simulink model "Wind_Turbine_MPPT_Simulation"  (R2023a)
settings: Solver=ode4  StartTime=0.0  StopTime=10  FixedStep=0.001  RelTol=1e-3
settings Model: Creator=32713  LastModifiedBy=32713

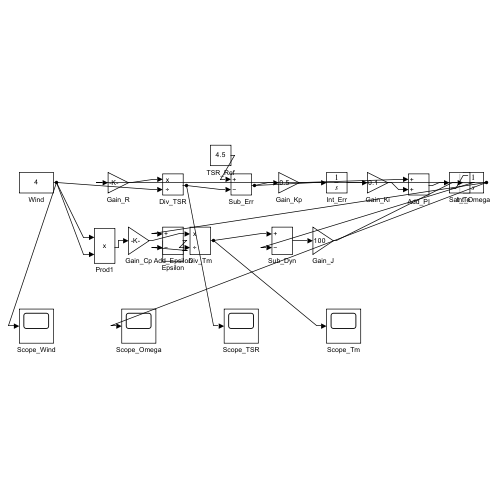
[thumbnail: Simulink's stored preview of the top-level diagram]
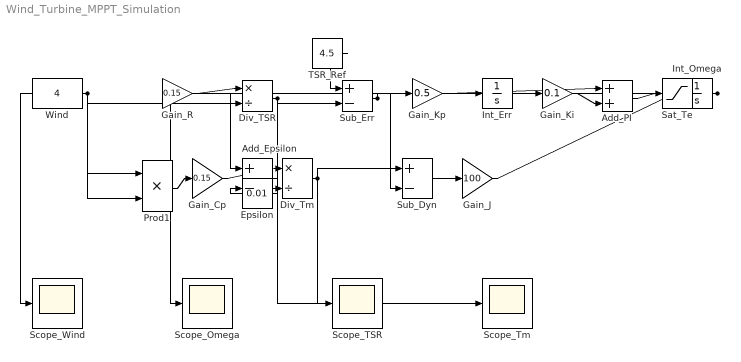
== system Wind_Turbine_MPPT_Simulation ==
  Add_Epsilon : Sum  Inputs=+-
  Add_PI : Sum
  Div_TSR : Product  Inputs=*/
  Div_Tm : Product  Inputs=*/
  Epsilon : Constant  Value=0.01
  Gain_Cp : Gain  Gain=0.15
  Gain_J : Gain  Gain=100
  Gain_Ki : Gain  Gain=0.1
  Gain_Kp : Gain  Gain=0.5
  Gain_R : Gain  Gain=0.15
  Int_Err : Integrator  InitialCondition=4.5
  Int_Omega : Integrator  InitialCondition=0.1
  Prod1 : Product
  Sat_Te : Saturate  UpperLimit=3  LowerLimit=0
  Scope_Omega : Scope
  Scope_TSR : Scope
  Scope_Tm : Scope
  Scope_Wind : Scope
  Sub_Dyn : Sum  Inputs=+-
  Sub_Err : Sum  Inputs=+-
  TSR_Ref : Constant  Value=4.5
  Wind : Constant  Value=4
  wires:
  Int_Omega/1 -> Gain_R/1, Add_Epsilon/1, Scope_Omega/1
  Gain_R/1 -> Div_TSR/1
  Wind/1 -> Div_TSR/2, Prod1/1, Prod1/2, Scope_Wind/1
  Div_TSR/1 -> Sub_Err/2, Scope_TSR/1
  TSR_Ref/1 -> Sub_Err/1
  Sub_Err/1 -> Gain_Kp/1, Int_Err/1
  Gain_Kp/1 -> Add_PI/1
  Int_Err/1 -> Gain_Ki/1
  Gain_Ki/1 -> Add_PI/2
  Add_PI/1 -> Sat_Te/1
  Sat_Te/1 -> Sub_Dyn/2
  Sub_Dyn/1 -> Gain_J/1
  Gain_J/1 -> Int_Omega/1
  Prod1/1 -> Gain_Cp/1
  Gain_Cp/1 -> Div_Tm/1
  Epsilon/1 -> Add_Epsilon/2
  Add_Epsilon/1 -> Div_Tm/2
  Div_Tm/1 -> Sub_Dyn/1, Scope_Tm/1
